simulink model "MATLAB_ROS_Manual"  (R2019b)
settings: Solver=FixedStepAuto  StartTime=0.0  StopTime=inf  FixedStep=0.01  RelTol=1e-3
undefined symbols (not defined in the file or in its folder): Brake, Steer, Throttle
libraries: robotlib x6, simulink x3, robotcorelib x1, simulink_extras x1, mpclib x1
settings Model: Creator=jiyo  LastModifiedBy=jiyo

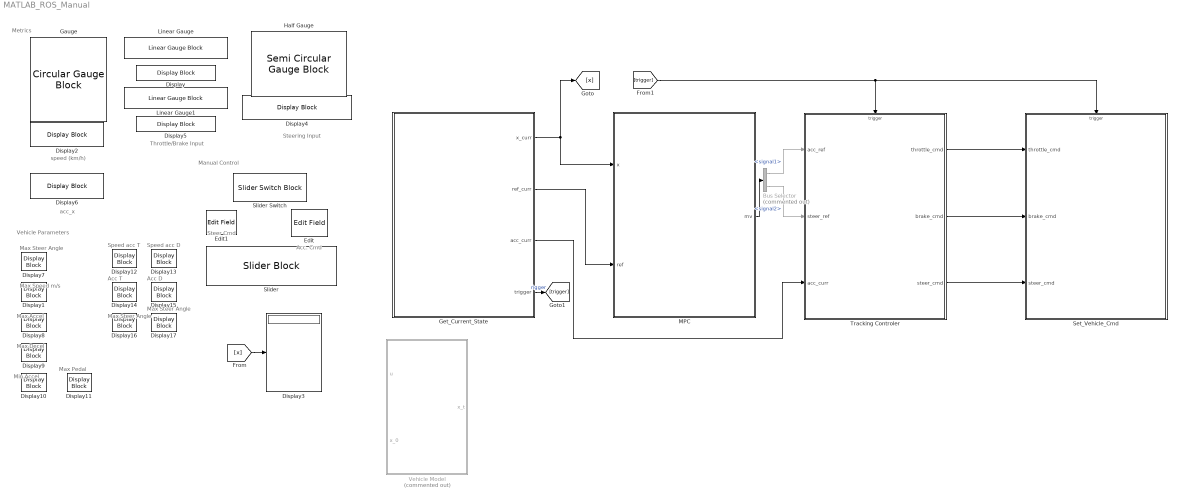
== system MATLAB_ROS_Manual ==
  note: speed (km/h)
  note: acc_x
  note: Acc. Cmd
  note: Steer Cmd
  note: Max Steer Angle
  note: Vehicle Parameters
  note: Throttle/Brake Input
  note: Manual Control
  note: Metrics
  note: Steering Input
  note: Max Speed m/s
  note: Max Accel
  note: Max Decel
  note: Min Accel
  note: Max Pedal
  note: Speed acc T
  note: Speed acc D
  note: Acc T
  note: Acc D
  note: Max Steer Angle
  note: Max Steer Angle
  Bus Selector : BusSelector  Commented=on  OutputSignals=signal1,signal2
  Display{,1..2,4..17} (17 alike) : DisplayBlock  LabelPosition=Hide  Format=short  Transparency=1
  Display3 : Display
  Edit : EditField  LabelPosition=Hide  ShowInitialText=on  Alignment=Center
  Edit1 : EditField  LabelPosition=Hide  ShowInitialText=on  Alignment=Center
  Gauge : CircularGaugeBlock  LabelPosition=Hide
  Get_Current_State : Subsystem
  Half Gauge : SemiCircularGaugeBlock  LabelPosition=Bottom  ScaleMin=-1  ScaleMax=1
  Linear Gauge : LinearGaugeBlock  LabelPosition=Bottom  ScaleMax=1
  Linear Gauge1 : LinearGaugeBlock  ScaleMax=1
  MPC : Subsystem
  Set_Vehicle_Cmd : Subsystem
  Slider : SliderBlock  LabelPosition=Bottom  ScaleMin=-1.571  ScaleMax=1.571
  Slider Switch : SliderSwitchBlock  LabelPosition=Bottom
      settings: Values={{'Off', 'On'}, [0 1]}
  Tracking Controler : Subsystem
  Vehicle Model : Subsystem  Commented=on
  wires:
  Get_Current_State/1(x_curr) -> [x], MPC/1(x)
  Get_Current_State/2(ref_curr) -> MPC/2(ref)
  [x] -> Display3/1
  MPC/1(mv) -> Bus Selector/1
  Tracking Controler/1(throttle_cmd) -> Set_Vehicle_Cmd/1(throttle_cmd)
  Tracking Controler/2(brake_cmd) -> Set_Vehicle_Cmd/2(brake_cmd)
  Tracking Controler/3(steer_cmd) -> Set_Vehicle_Cmd/3(steer_cmd)
  Get_Current_State/3(acc_curr) -> Tracking Controler/3(acc_curr)
  Bus Selector/1 -> Tracking Controler/1(acc_ref)  "<signal1>"
  Bus Selector/2 -> Tracking Controler/2(steer_ref)  "<signal2>"
  Get_Current_State/4(trigger) -> [trigger]  "rigger"
  [trigger] -> Set_Vehicle_Cmd/Trigger, Tracking Controler/Trigger

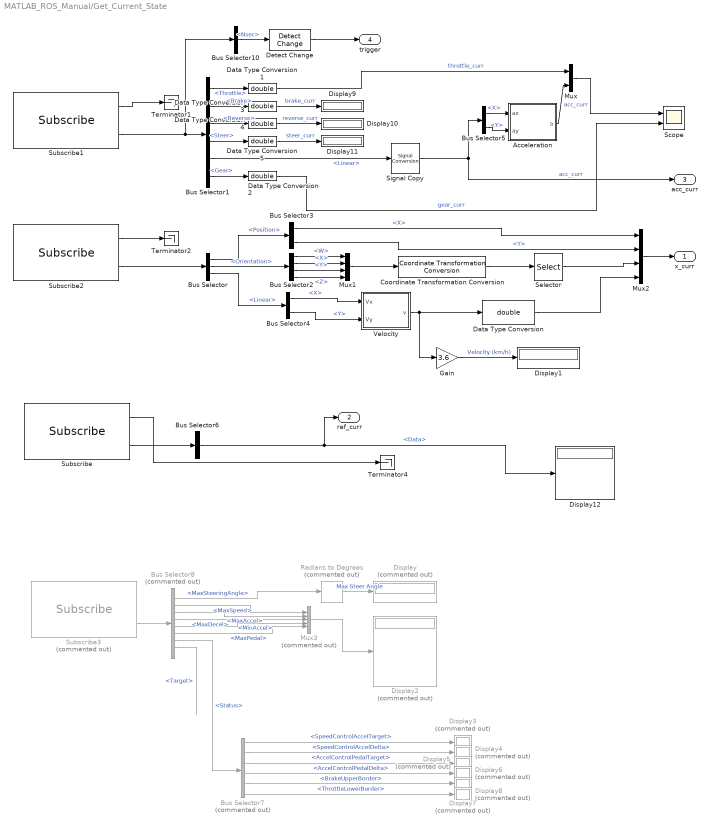
== system MATLAB_ROS_Manual/Get_Current_State ==
  Acceleration : Subsystem
  Bus Selector : BusSelector  OutputSignals=Pose.Pose.Position,Pose.Pose.Orientation,Twist.Twist.Linear
  Bus Selector1 : BusSelector  OutputSignals=Control.Throttle,Control.Brake,Control.Reverse,Control.Steer,Acceleration.Linear,Control.Gear
  Bus Selector10 : BusSelector  OutputSignals=Header.Stamp.Nsec
  Bus Selector2 : BusSelector  OutputSignals=W,X,Y,Z
  Bus Selector3 : BusSelector  OutputSignals=X,Y
  Bus Selector4 : BusSelector  OutputSignals=X,Y
  Bus Selector5 : BusSelector  OutputSignals=X,Y
  Bus Selector6 : BusSelector  OutputSignals=Data
  Bus Selector7 : BusSelector  Commented=on  OutputSignals=SpeedControlAccelTarget,SpeedControlAccelDelta,AccelControlPedalTarget,AccelControlPedalDelta,BrakeUpperBorder,ThrottleLowerBorder
  Bus Selector8 : BusSelector  Commented=on  OutputSignals=Restrictions.MaxSteeringAngle,Restrictions.MaxSpeed,Restrictions.MaxAccel,Restrictions.MaxDecel,Restrictions.MinAccel,Restrictions.MaxPedal,Status,Target
  Coordinate Transformation Conversion : robotcorelib/Coordinate Transformation Conversion  InputRepresentation=Quaternion  InputEulerSequence=ZYX  ShowTrVecInputPort=on  OutputRepresentation=Euler Angles  OutputEulerSequence=ZYX  ShowTrVecOutputPort=on  SimulateUsing=Interpreted execution
      settings: SourceProductBaseCode=RO
  Data Type Conversion{,1..5} (6 alike) : DataTypeConversion  OutDataTypeStr=double
  Detect Change : simulink/Logic and Bit Operations/Detect Change  vinit=0  OutDataTypeStr=boolean
  Display{,2..8} (8 alike) : Display  Commented=on
  Display{1,9..12} (5 alike) : Display
  Gain : Gain  Gain=3.6
  Mux : Mux  Inputs=2
  Mux1 : Mux
  Mux2 : Mux
  Mux3 : Mux  Commented=on  Inputs=5
  Radians to Degrees : simulink_extras/Transformations/Radians to Degrees  Commented=on
  Scope : Scope  NumInputPorts=2
  Selector : Selector  InputPortWidth=3  IndexOptions=Index vector (dialog)  Indices=[1]  OutputSizes=1
  Signal Copy : SignalConversion  ConversionOutput=Virtual bus  OverrideOpt=off
  Subscribe : robotlib/Subscribe  topicSource=Select from ROS network  topic=/X_Ref  messageType=custom_msgs/Float64Arr4  sampleTime=-1  messageQueueLength=1
      settings: SourceProductName=ROS Toolbox
  Subscribe1 : robotlib/Subscribe  topicSource=Select from ROS network  topic=/carla/ego_vehicle/vehicle_status  messageType=carla_msgs/CarlaEgoVehicleStatus  sampleTime=-1  messageQueueLength=1
      settings: SourceProductName=ROS Toolbox
  Subscribe2 : robotlib/Subscribe  topicSource=Select from ROS network  topic=/carla/ego_vehicle/odometry  messageType=nav_msgs/Odometry  sampleTime=-1  messageQueueLength=1
      settings: SourceProductName=ROS Toolbox
  Subscribe3 : robotlib/Subscribe  Commented=on  topicSource=Select from ROS network  topic=/carla/ego_vehicle/ackermann_control/control_info  messageType=carla_ackermann_control/EgoVehicleControlInfo  sampleTime=-1  messageQueueLength=1
      settings: SourceProductName=ROS Toolbox
  Terminator1 : Terminator
  Terminator2 : Terminator
  Terminator4 : Terminator
  Velocity : Subsystem
  x_curr : Outport
  ref_curr : Outport  Port=2
  acc_curr : Outport  Port=3
  trigger : Outport  Port=4
  wires:
  Subscribe1/2 -> Bus Selector10/1, Bus Selector1/1
  Bus Selector1/1 -> Data Type Conversion1/1  "<Throttle>"
  Bus Selector/2 -> Bus Selector2/1  "<Orientation>"
  Subscribe2/2 -> Bus Selector/1
  Bus Selector1/4 -> Data Type Conversion5/1  "<Steer>"
  Bus Selector2/4 -> Mux1/4  "<Z>"
  Bus Selector/1 -> Bus Selector3/1  "<Position>"
  Bus Selector2/1 -> Mux1/1  "<W>"
  Coordinate Transformation Conversion/1 -> Selector/1
  Subscribe2/1 -> Terminator2/1
  Bus Selector1/3 -> Data Type Conversion4/1  "<Reverse>"
  Bus Selector3/2 -> Mux2/2  "<Y>"
  Bus Selector2/3 -> Mux1/3  "<Y>"
  Data Type Conversion/1 -> Mux2/4
  Mux1/1 -> Coordinate Transformation Conversion/1
  Gain/1 -> Display1/1  "Velocity (km/h)"
  Bus Selector/3 -> Bus Selector4/1  "<Linear>"
  Velocity/1(v) -> Gain/1, Data Type Conversion/1
  Bus Selector2/2 -> Mux1/2  "<X>"
  Bus Selector4/2 -> Velocity/2(Vy)  "<Y>"
  Bus Selector3/1 -> Mux2/1  "<X>"
  Selector/1 -> Mux2/3
  Bus Selector4/1 -> Velocity/1(Vx)  "<X>"
  Mux2/1 -> x_curr/1
  Subscribe1/1 -> Terminator1/1
  Subscribe/1 -> Terminator4/1
  Bus Selector1/5 -> Signal Copy/1  "<Linear>"
  Mux/1 -> Scope/1
  Data Type Conversion1/1 -> Mux/1  "throttle_curr"
  Bus Selector1/6 -> Data Type Conversion2/1  "<Gear>"
  Data Type Conversion2/1 -> Scope/2  "gear_curr"
  Radians to Degrees/1 -> Display/1  "Max Steer Angle"
  Bus Selector1/2 -> Data Type Conversion3/1  "<Brake>"
  Subscribe3/2 -> Bus Selector8/1
  Bus Selector8/1 -> Radians to Degrees/1  "<MaxSteeringAngle>"
  Bus Selector8/2 -> Mux3/1  "<MaxSpeed>"
  Bus Selector8/3 -> Mux3/2  "<MaxAccel>"
  Bus Selector8/4 -> Mux3/3  "<MaxDecel>"
  Bus Selector8/5 -> Mux3/4  "<MinAccel>"
  Bus Selector8/6 -> Mux3/5  "<MaxPedal>"
  Bus Selector8/7 -> Bus Selector7/1  "<Status>"
  Bus Selector8/8 -> ?  "<Target>"
  Mux3/1 -> Display2/1
  Bus Selector7/1 -> Display3/1  "<SpeedControlAccelTarget>"
  Bus Selector7/2 -> Display4/1  "<SpeedControlAccelDelta>"
  Bus Selector7/3 -> Display5/1  "<AccelControlPedalTarget>"
  Bus Selector7/4 -> Display6/1  "<AccelControlPedalDelta>"
  Bus Selector7/5 -> Display7/1  "<BrakeUpperBorder>"
  Bus Selector7/6 -> Display8/1  "<ThrottleLowerBorder>"
  Signal Copy/1 -> Bus Selector5/1, acc_curr/1  "acc_curr"
  Bus Selector5/1 -> Acceleration/1(ax)  "<X>"
  Bus Selector5/2 -> Acceleration/2(ay)  "<Y>"
  Acceleration/1(a) -> Mux/2  "acc_curr"
  Data Type Conversion3/1 -> Display9/1  "brake_curr"
  Data Type Conversion4/1 -> Display10/1  "reverse_curr"
  Data Type Conversion5/1 -> Display11/1  "steer_curr"
  Bus Selector10/1 -> Detect Change/1  "<Nsec>"
  Detect Change/1 -> trigger/1
  Bus Selector6/1 -> ref_curr/1, Display12/1  "<Data>"
  Subscribe/2 -> Bus Selector6/1

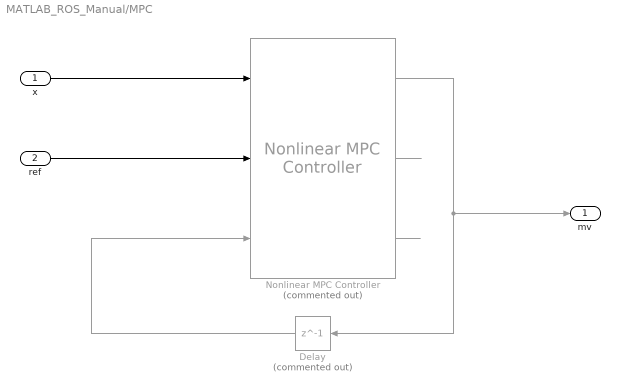
== system MATLAB_ROS_Manual/MPC ==
  x : Inport
  ref : Inport  Port=2
  Delay : Delay  Commented=on  DelayLength=1
  Nonlinear MPC Controller : mpclib/Nonlinear MPC Controller  Commented=on  SCDEnableBlockLinearizationSpecification=on  UseObjectTs=on  md_enabled=off  mvtarget_enabled=off  param_enabled=off  cost_enabled=off  mvseq_enabled=on  stateseq_enabled=off  ovseq_enabled=on  slack_enabled=off  status_enabled=off  ov_min=off  ov_max=off  mv_min=off  mv_max=off  mvrate_min=off  mvrate_max=off  state_min=off  state_max=off  ov_weight=off  mv_weight=off  mvrate_weight=off  ecr_weight=off  nlp_initialize=off
      settings: SourceProductName=Model Predictive Control Toolbox
  mv : Outport
  wires:
  Nonlinear MPC Controller/1 -> Delay/1, mv/1
  x/1 -> Nonlinear MPC Controller/1
  ref/1 -> Nonlinear MPC Controller/2
  Delay/1 -> Nonlinear MPC Controller/3
  Nonlinear MPC Controller/2 -> ?
  Nonlinear MPC Controller/3 -> ?

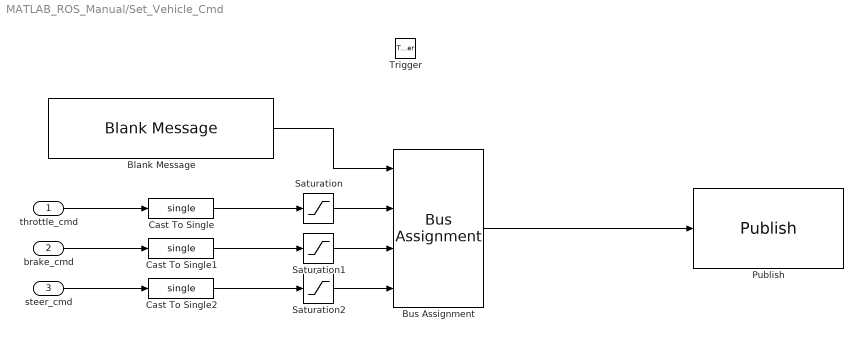
== system MATLAB_ROS_Manual/Set_Vehicle_Cmd ==
  throttle_cmd : Inport
  brake_cmd : Inport  Port=2
  steer_cmd : Inport  Port=3
  Trigger : TriggerPort  VariantControl=Variant  PortDimensions=1
  Blank Message : robotlib/Blank Message  messageClass=Message  entityType=carla_msgs/CarlaEgoVehicleControl  messageType=carla_msgs/CarlaEgoVehicleControl  SampleTime=inf
      settings: SourceProductName=ROS Toolbox
  Bus Assignment : BusAssignment  AssignedSignals=Throttle,Brake,Steer
  Cast To Single : DataTypeConversion  OutDataTypeStr=single
  Cast To Single1 : DataTypeConversion  OutDataTypeStr=single
  Cast To Single2 : DataTypeConversion  OutDataTypeStr=single
  Publish : robotlib/Publish  topicSource=Select from ROS network  topic=/carla/ego_vehicle/vehicle_control_cmd  messageType=carla_msgs/CarlaEgoVehicleControl  messageQueueLength=1
      settings: SourceProductName=ROS Toolbox
  Saturation : Saturate  UpperLimit=1  LowerLimit=0
  Saturation1 : Saturate  UpperLimit=1  LowerLimit=0
  Saturation2 : Saturate  UpperLimit=1  LowerLimit=-1
  wires:
  Blank Message/1 -> Bus Assignment/1
  Bus Assignment/1 -> Publish/1
  steer_cmd/1 -> Cast To Single2/1
  brake_cmd/1 -> Cast To Single1/1
  throttle_cmd/1 -> Cast To Single/1
  Saturation/1 -> Bus Assignment/2
  Saturation1/1 -> Bus Assignment/3
  Saturation2/1 -> Bus Assignment/4
  Cast To Single/1 -> Saturation/1
  Cast To Single1/1 -> Saturation1/1
  Cast To Single2/1 -> Saturation2/1

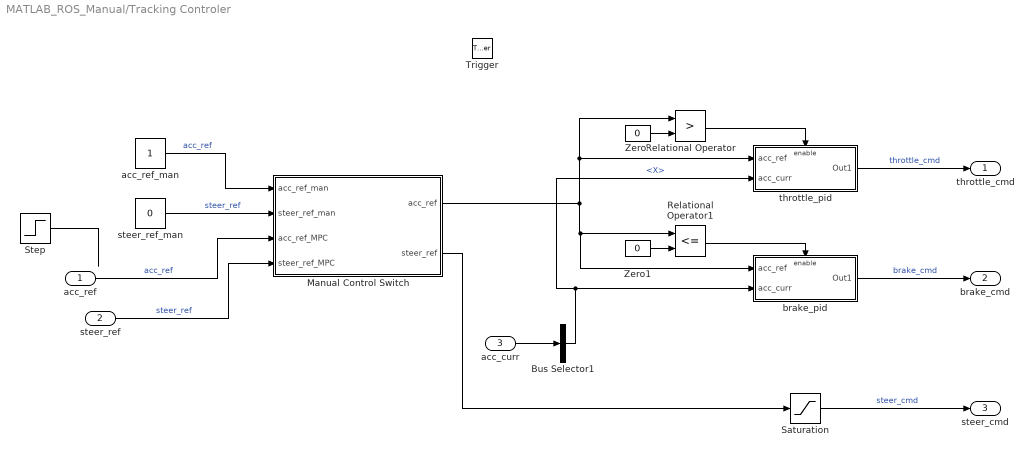
== system MATLAB_ROS_Manual/Tracking Controler ==
  acc_ref : Inport
  steer_ref : Inport  Port=2
  acc_curr : Inport  Port=3
  Trigger : TriggerPort  VariantControl=Variant  PortDimensions=1
  Bus Selector1 : BusSelector  OutputSignals=X
  Manual Control Switch : Subsystem
  Relational Operator : RelationalOperator  Operator=>  OutDataTypeStr=boolean  RndMeth=Simplest
  Relational Operator1 : RelationalOperator  Operator=<=  OutDataTypeStr=boolean  RndMeth=Simplest
  Saturation : Saturate  UpperLimit=1  LowerLimit=-1
  Step : Step  After=2  SampleTime=0
  Zero : Constant  Value=0  OutDataTypeStr=Inherit: Inherit via back propagation
  Zero1 : Constant  Value=0  OutDataTypeStr=Inherit: Inherit via back propagation
  acc_ref_man : Constant
  brake_pid : Subsystem  TreatAsAtomicUnit=on
  steer_ref_man : Constant  Value=0
  throttle_pid : Subsystem  TreatAsAtomicUnit=on
  throttle_cmd : Outport
  brake_cmd : Outport  Port=2
  steer_cmd : Outport  Port=3
  wires:
  Bus Selector1/1 -> throttle_pid/2(acc_curr), brake_pid/2(acc_curr)  "<X>"
  throttle_pid/1(Out1) -> throttle_cmd/1  "throttle_cmd"
  brake_pid/1(Out1) -> brake_cmd/1  "brake_cmd"
  Relational Operator/1 -> throttle_pid/Enable
  Zero/1 -> Relational Operator/2
  Zero1/1 -> Relational Operator1/2
  Relational Operator1/1 -> brake_pid/Enable
  Saturation/1 -> steer_cmd/1  "steer_cmd"
  acc_curr/1 -> Bus Selector1/1
  Manual Control Switch/1(acc_ref) -> brake_pid/1(acc_ref), Relational Operator1/1, throttle_pid/1(acc_ref), Relational Operator/1
  acc_ref_man/1 -> Manual Control Switch/1(acc_ref_man)  "acc_ref"
  steer_ref_man/1 -> Manual Control Switch/2(steer_ref_man)  "steer_ref"
  acc_ref/1 -> Manual Control Switch/3(acc_ref_MPC)  "acc_ref"
  steer_ref/1 -> Manual Control Switch/4(steer_ref_MPC)  "steer_ref"
  Manual Control Switch/2(steer_ref) -> Saturation/1
  Step/1 -> ?

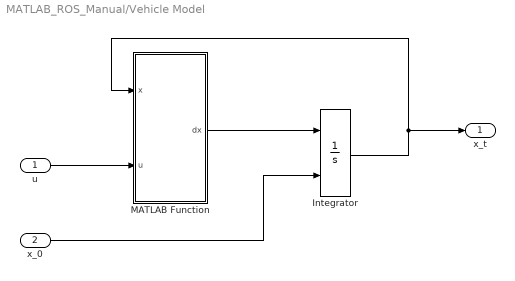
== system MATLAB_ROS_Manual/Vehicle Model ==
  u : Inport
  x_0 : Inport  Port=2
  Integrator : Integrator  InitialConditionSource=external
  MATLAB Function : MATLAB Function  TreatAsAtomicUnit=on
  x_t : Outport
  wires:
  u/1 -> MATLAB Function/2(u)
  MATLAB Function/1(dx) -> Integrator/1
  Integrator/1 -> MATLAB Function/1(x), x_t/1
  x_0/1 -> Integrator/2

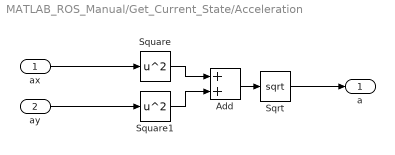
== system MATLAB_ROS_Manual/Get_Current_State/Acceleration ==
  ax : Inport
  ay : Inport  Port=2
  Add : Sum
  Sqrt : Sqrt  SaturateOnIntegerOverflow=on
  Square : Math  Operator=square  SignedPower=off  SaturateOnIntegerOverflow=on
  Square1 : Math  Operator=square  SignedPower=off  SaturateOnIntegerOverflow=on
  a : Outport
  wires:
  Square/1 -> Add/1
  Add/1 -> Sqrt/1
  Square1/1 -> Add/2
  Sqrt/1 -> a/1
  ax/1 -> Square/1
  ay/1 -> Square1/1

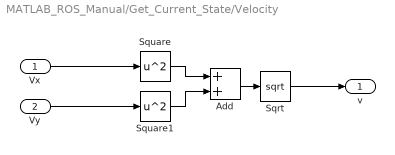
== system MATLAB_ROS_Manual/Get_Current_State/Velocity ==
  Vx : Inport
  Vy : Inport  Port=2
  Add : Sum
  Sqrt : Sqrt  SaturateOnIntegerOverflow=on
  Square : Math  Operator=square  SignedPower=off  SaturateOnIntegerOverflow=on
  Square1 : Math  Operator=square  SignedPower=off  SaturateOnIntegerOverflow=on
  v : Outport
  wires:
  Vy/1 -> Square1/1
  Vx/1 -> Square/1
  Sqrt/1 -> v/1
  Square1/1 -> Add/2
  Add/1 -> Sqrt/1
  Square/1 -> Add/1

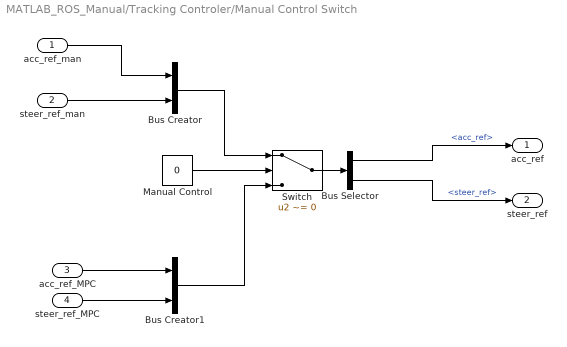
== system MATLAB_ROS_Manual/Tracking Controler/Manual Control Switch ==
  acc_ref_man : Inport
  steer_ref_man : Inport  Port=2
  acc_ref_MPC : Inport  Port=3
  steer_ref_MPC : Inport  Port=4
  Bus Creator : BusCreator  Inputs=2
  Bus Creator1 : BusCreator  Inputs=2
  Bus Selector : BusSelector  OutputSignals=acc_ref,steer_ref
  Manual Control : Constant  Value=0  OutDataTypeStr=boolean
  Switch : Switch  Criteria=u2 ~= 0
  acc_ref : Outport
  steer_ref : Outport  Port=2
  wires:
  Bus Selector/2 -> steer_ref/1  "<steer_ref>"
  Bus Creator/1 -> Switch/1
  acc_ref_man/1 -> Bus Creator/1
  steer_ref_man/1 -> Bus Creator/2
  steer_ref_MPC/1 -> Bus Creator1/2
  Manual Control/1 -> Switch/2
  acc_ref_MPC/1 -> Bus Creator1/1
  Bus Creator1/1 -> Switch/3
  Bus Selector/1 -> acc_ref/1  "<acc_ref>"
  Switch/1 -> Bus Selector/1

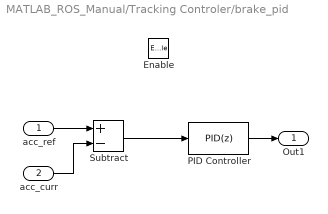
== system MATLAB_ROS_Manual/Tracking Controler/brake_pid ==
  acc_ref : Inport
  acc_curr : Inport  Port=2
  Enable : EnablePort
  PID Controller : simulink/Continuous/PID Controller  Controller=PID  Form=Parallel  TimeDomain=Discrete-time  SampleTime=-1  IntegratorMethod=Forward Euler  FilterMethod=Forward Euler  ControllerParametersSource=internal  P=1  I=1  D=0  UseFilter=on  N=100  TunerSelectOption=Transfer Function Based (PID Tuner App)  InitialConditionSource=internal  InitialConditionForIntegrator=0  InitialConditionForFilter=0  DifferentiatorICPrevScaledInput=0  ExternalReset=none  TrackingMode=off  Kt=1  LimitOutput=on  UpperSaturationLimit=1  LowerSaturationLimit=0  LinearizeAsGain=on  AntiWindupMode=none  Kb=1  POutMin=[]  POutMax=[]  IOutMin=[]  IOutMax=[]  DOutMin=[]  DOutMax=[]  NOutMin=[]  NOutMax=[]  SumOutMin=[]  SumOutMax=[]  SaturationOutMin=[]  SaturationOutMax=[]  PParamMin=[]  PParamMax=[]  IParamMin=[]  IParamMax=[]  DParamMin=[]  DParamMax=[]  NParamMin=[]  NParamMax=[]  KbParamMin=[]  KbParamMax=[]  KtParamMin=[]  KtParamMax=[]  KbOutMin=[]  KbOutMax=[]  KtOutMin=[]  KtOutMax=[]  IntegratorOutMin=[]  IntegratorOutMax=[]  FilterOutMin=[]  FilterOutMax=[]  SumI1OutMin=[]  SumI1OutMax=[]  SumI2OutMin=[]  SumI2OutMax=[]  SumI3OutMin=[]  SumI3OutMax=[]  SumI4OutMin=[]  SumI4OutMax=[]  SumDOutMin=[]  SumDOutMax=[]  DifferentiatorOutMin=[]  DifferentiatorOutMax=[]  FilterDiffOutCoefMin=[]  FilterDiffOutCoefMax=[]  ReciprocalOutMin=[]  ReciprocalOutMax=[]  SumDenOutMin=[]  SumDenOutMax=[]  SumNumOutMin=[]  SumNumOutMax=[]  DivideOutMin=[]  DivideOutMax=[]  IntegratorContinuousStateAttributes=''  IntegratorStateMustResolveToSignalObject=off  IntegratorRTWStateStorageClass=Auto  FilterContinuousStateAttributes=''  FilterStateMustResolveToSignalObject=off  FilterRTWStateStorageClass=Auto  ParallelPVariant=InternalParameters  IdealPVariant=Disabled  IVariant=InternalParameters  DVariant=InternalParameters  IntegratorVariant=Discrete  SatVariant=Enabled  AWVariant=Passthrough  PCopyVariant=Disabled  TRVariant=Disabled  FdbkBlocksVariant=Forward  IdealPFdbkVariant=Disabled  SatFdbkVariant=Disabled  DerivativeFilterVariant=ForwardEulerFilter  NVariant=InternalParameters  NCopyVariant=Disabled  FilterICVariant=InternalICsFilter  IntegratorICVariant=InternalICs  ExternalResetVariant=Disabled  TRSumVariant=Passthrough  SumFdbkVariant=Disabled  SumVariant=Sum_PID
  Subtract : Sum  Inputs=+-
  Out1 : Outport
  wires:
  Subtract/1 -> PID Controller/1
  acc_curr/1 -> Subtract/2
  PID Controller/1 -> Out1/1
  acc_ref/1 -> Subtract/1

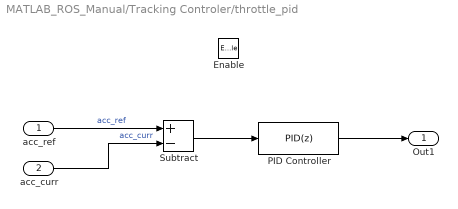
== system MATLAB_ROS_Manual/Tracking Controler/throttle_pid ==
  acc_ref : Inport
  acc_curr : Inport  Port=2
  Enable : EnablePort
  PID Controller : simulink/Continuous/PID Controller  Controller=PID  Form=Parallel  TimeDomain=Discrete-time  SampleTime=-1  IntegratorMethod=Forward Euler  FilterMethod=Forward Euler  ControllerParametersSource=internal  P=0.15  I=0.1  D=0  UseFilter=on  N=100  TunerSelectOption=Transfer Function Based (PID Tuner App)  InitialConditionSource=internal  InitialConditionForIntegrator=0  InitialConditionForFilter=0  DifferentiatorICPrevScaledInput=0  ExternalReset=none  TrackingMode=off  Kt=1  LimitOutput=on  UpperSaturationLimit=1  LowerSaturationLimit=0  LinearizeAsGain=on  AntiWindupMode=none  Kb=1  POutMin=[]  POutMax=[]  IOutMin=[]  IOutMax=[]  DOutMin=[]  DOutMax=[]  NOutMin=[]  NOutMax=[]  SumOutMin=[]  SumOutMax=[]  SaturationOutMin=[]  SaturationOutMax=[]  PParamMin=[]  PParamMax=[]  IParamMin=[]  IParamMax=[]  DParamMin=[]  DParamMax=[]  NParamMin=[]  NParamMax=[]  KbParamMin=[]  KbParamMax=[]  KtParamMin=[]  KtParamMax=[]  KbOutMin=[]  KbOutMax=[]  KtOutMin=[]  KtOutMax=[]  IntegratorOutMin=[]  IntegratorOutMax=[]  FilterOutMin=[]  FilterOutMax=[]  SumI1OutMin=[]  SumI1OutMax=[]  SumI2OutMin=[]  SumI2OutMax=[]  SumI3OutMin=[]  SumI3OutMax=[]  SumI4OutMin=[]  SumI4OutMax=[]  SumDOutMin=[]  SumDOutMax=[]  DifferentiatorOutMin=[]  DifferentiatorOutMax=[]  FilterDiffOutCoefMin=[]  FilterDiffOutCoefMax=[]  ReciprocalOutMin=[]  ReciprocalOutMax=[]  SumDenOutMin=[]  SumDenOutMax=[]  SumNumOutMin=[]  SumNumOutMax=[]  DivideOutMin=[]  DivideOutMax=[]  IntegratorContinuousStateAttributes=''  IntegratorStateMustResolveToSignalObject=off  IntegratorRTWStateStorageClass=Auto  FilterContinuousStateAttributes=''  FilterStateMustResolveToSignalObject=off  FilterRTWStateStorageClass=Auto  ParallelPVariant=InternalParameters  IdealPVariant=Disabled  IVariant=InternalParameters  DVariant=InternalParameters  IntegratorVariant=Discrete  SatVariant=Enabled  AWVariant=Passthrough  PCopyVariant=Disabled  TRVariant=Disabled  FdbkBlocksVariant=Forward  IdealPFdbkVariant=Disabled  SatFdbkVariant=Disabled  DerivativeFilterVariant=ForwardEulerFilter  NVariant=InternalParameters  NCopyVariant=Disabled  FilterICVariant=InternalICsFilter  IntegratorICVariant=InternalICs  ExternalResetVariant=Disabled  TRSumVariant=Passthrough  SumFdbkVariant=Disabled  SumVariant=Sum_PID
  Subtract : Sum  Inputs=+-
  Out1 : Outport
  wires:
  acc_ref/1 -> Subtract/1  "acc_ref"
  PID Controller/1 -> Out1/1
  acc_curr/1 -> Subtract/2  "acc_curr"
  Subtract/1 -> PID Controller/1

== matlab function MATLAB_ROS_Manual/Vehicle Model/MATLAB Function ==
  data: x input; u input; dx output
function dx = fcn(x,u)
dx = vkinematicmodel_bicycle(x,u);
